simulink model "nmm2DFullBody"  (R2015b)
settings: Solver=ode23s  StartTime=0.0  StopTime=13  FixedStep=1e-3  MaxStep=ts_max  RelTol=1e-3  AbsTol=1e-4
InitFcn:
  | addpath('../lib');
  | addpath('./init_script');
  | nms_model_MechInit
  | nms_model_ControlInit
StopFcn:
  | mRFX = struct;
  | 
  | mRFX.RStance = DataFromModel.Data(:,2)
  | mRFX.RGRF_AP = DataFromModel.Data(:,24)
  | mRFX.RGRF_VT = DataFromModel.Data(:,22)
  | mRFX.RAnkleAngle = DataFromModel.Data(:,8)
  | mRFX.RKneeAngle = DataFromModel.Data(:,7)
  | mRFX.RHipAngle = DataFromModel.Data(:,6)
  | mRFX.RAnkleTorque = DataFromModel.Data(:,20)
  | mRFX.RKneeTorque = DataFromModel.Data(:,19)
  | mRFX.RHipTorque = DataFromModel.Data(:,18)
  | 
  | mRFX.RMuscleGLU = DataFromModel.Data(:,32)
  | mRFX.RMuscleHF = DataFromModel.Data(:,33)
  | mRFX.RMuscleHAM = DataFromModel.Data(:,34)
  | mRFX.RMuscleVAS = DataFromModel.Data(:,35)
  | mRFX.RMuscleGAS = DataFromModel.Data(:,36)
  | mRFX.RMuscleSOL = DataFromModel.Data(:,37)
  | mRFX.RMuscleTA = DataFromModel.Data(:,38)
  | 
  | mRFX.LStance = DataFromModel.Data(:,1)
  | mRFX.LGRF_AP = DataFromModel.Data(:,23)
  | mRFX.LGRF_VT = DataFromModel.Data(:,21)
  | mRFX.LAnkleAngle = DataFromModel.Data(:,5)
  | mRFX.LKneeAngle = DataFromModel.Data(:,4)
  | mRFX.LHipAngle = DataFromModel.Data(:,3)
  | mRFX.LAnkleTorque = DataFromModel.Data(:,17)
  | mRFX.LKneeTorque = DataFromModel.Data(:,16)
  | mRFX.LHipTorque = DataFromModel.Data(:,15)
  | 
  | mRFX.LMuscleGLU = DataFromModel.Data(:,25)
  | mRFX.LMuscleHF = DataFromModel.Data(:,26)
  | mRFX.LMuscleHAM = DataFromModel.Data(:,27)
  | mRFX.LMuscleVAS = DataFromModel.Data(:,28)
  | mRFX.LMuscleGAS = DataFromModel.Data(:,29)
  | mRFX.LMuscleSOL = DataFromModel.Data(:,30)
  | mRFX.LMuscleTA = DataFromModel.Data(:,31)
values from neighbouring files (symbols this model uses):
  c = load('struct_mRFX_HAM_symetric_feedback.mat')    [Ex2b.m]
undefined symbols (not defined in the file or in its folder): alphaFmGas, alphaFmGlu, alphaFmHam, alphaFmSol, alphaFmVas, alphaLceHam, alphaLceHfl, alphaLceTa, alphaLceTa1, Amp, amp_var, c_jointstop, D12_F, D12_S, D12_T, D13_F, D1G_F, D1G_HAT, D1G_S, D1G_T, DeltaThRef, eref, FmaxGAS, FmaxGLU, FmaxHAM, FmaxHFL, FmaxSOL, FmaxTA, FmaxVAS, freq, freq_var, GainDeltaTheta, GainGAS, GainGLU, GainHAM, GainHAMHFL, GainHFL, GainKneOverExt, GainSOL, GainSOLTA, GainTA, GainVAS, In_F, In_HAT, In_S, In_T, K, k_gx, k_gy, k_pressure, K_swing, LceOffsetHAM, LceOffsetHFL, LceOffsetTA, LongDelay, loptGAS, loptGLU, loptHAM, loptHFL, loptSOL ... (+82)
libraries: nmc x77, mblibv1 x60, simulink x33, simulink_extras x18
(part 2 of 8)

== system nmm2DFullBody/Body Mechanics Layer (from Geyer s 2010 model)/Left Ball Contact ==
  note: Planar Ground Interaction Model
  Body Actuator : mblibv1/Sensors &  Actuators/Body Actuator  UpdateFromCAD=off  PhysicalDomain=Mechanical  PortType=blob  ActuationStyle=Force  AngleUnits=deg  ArcVelocityUnits=deg/s  ArcAccelerationUnits=deg/s^2  CoordPositionUnits=m  VelocityUnits=m/s  AccelerationUnits=m/s^2  ForceUnits=N  TorqueUnits=N-m  ActiveIO=on  Width=3  DialogClass=MechanicalActuatorBlock  ReferenceFrame=Absolute (World)  Angle=off  CoordPosition=on  Force=on  Torque=off
  Body Sensor : mblibv1/Sensors &  Actuators/Body Sensor  UpdateFromCAD=off  PhysicalDomain=Mechanical  PortType=blob  Muxed=on  Pose=off  Angle=on  AngleUnits=deg  ArcVelocity=off  ArcVelocityUnits=deg/s  ArcAcceleration=off  ArcAccelerationUnits=deg/s^2  CoordPosition=on  CoordPositionUnits=m  Velocity=on  VelocityUnits=m/s  Acceleration=off  AccelerationUnits=m/s^2  Quaternion=on  QuaternionDT=off  QuaternionDDT=off  QuaternionUnits=off  OutputVector=[ 3 3 ]  ActiveIO=on  Width=6  DialogClass=MechanicalSensorBlock  ReferenceFrame=Absolute (World)
  Demux1 : Demux
  Ground Friction Model : Subsystem
  Ground1 : Ground
  Mechanical Branching Bar : mblibv1/Utilities/Mechanical Branching Bar  LConnTagsString=_newl0  RConnTagsString=SA0|SA1  UpdateFromCAD=off  DialogClass=MechanicalBranchingBarBlock  NumSAPorts=2
  Mux : Mux  Inputs=2
  Mux1 : Mux  Inputs=3
  Sum : Sum  Inputs=-+|
  Terminator : Terminator
  To Workspace : ToWorkspace  VariableName=L_dyvyxvx  SaveFormat=Timeseries  SampleTime=-1
  Vector ConcatenateKnee : Concatenate  NumInputs=4
  "[y y' x x']" : Selector  InputPortWidth=6  IndexOptions=Index vector (dialog)  Indices=[2 5 1 4]  OutputSizes=1
  contact? : simulink/Logic and Bit Operations/Compare To Zero  relop=<=  OutDataTypeStr=boolean
  yGround : Constant  Value=0
  F : PMIOPort  Port=1  Side=Left
  LBallCnt : Outport
  GRF [N N] : Outport  Port=2
  wires:
  contact?/1 -> Ground Friction Model/Enable, LBallCnt/1
  Ground Friction Model/1(Fy_Ground[N]) -> Mux/2, Mux1/2
  Ground Friction Model/2(Fx_Friction [N]) -> Mux/1, Mux1/1
  Ground Friction Model/3(Stiction!) -> Terminator/1
  Mux/1 -> GRF [N N]/1
  yGround/1 -> Sum/1
  Sum/1 -> Vector ConcatenateKnee/1, Ground Friction Model/1(dy [m]), contact?/1
  Body Sensor/1 -> "[y y' x x']"/1
  Mux1/1 -> Body Actuator/1
  Demux1/1 -> Sum/2
  Demux1/2 -> Vector ConcatenateKnee/2, Ground Friction Model/2(vy [m/s])
  Demux1/4 -> Vector ConcatenateKnee/4, Ground Friction Model/4(vx [m/s])
  "[y y' x x']"/1 -> Demux1/1
  Ground1/1 -> Mux1/3
  Vector ConcatenateKnee/1 -> To Workspace/1
  Demux1/3 -> Vector ConcatenateKnee/3, Ground Friction Model/3(x [m])
  connections:
  F/RConn1 -- Mechanical Branching Bar/LConn1
  Mechanical Branching Bar/RConn1 -- Body Sensor/LConn1
  Mechanical Branching Bar/RConn2 -- Body Actuator/RConn1

== system nmm2DFullBody/Body Mechanics Layer (from Geyer s 2010 model)/Left Heel Contact ==
  note: Planar Ground Interaction Model
  Body Actuator : mblibv1/Sensors &  Actuators/Body Actuator  UpdateFromCAD=off  PhysicalDomain=Mechanical  PortType=blob  ActuationStyle=Force  AngleUnits=deg  ArcVelocityUnits=deg/s  ArcAccelerationUnits=deg/s^2  CoordPositionUnits=m  VelocityUnits=m/s  AccelerationUnits=m/s^2  ForceUnits=N  TorqueUnits=N-m  ActiveIO=on  Width=3  DialogClass=MechanicalActuatorBlock  ReferenceFrame=Absolute (World)  Angle=off  CoordPosition=on  Force=on  Torque=off
  Body Sensor : mblibv1/Sensors &  Actuators/Body Sensor  UpdateFromCAD=off  PhysicalDomain=Mechanical  PortType=blob  Muxed=on  Pose=off  Angle=on  AngleUnits=deg  ArcVelocity=off  ArcVelocityUnits=deg/s  ArcAcceleration=off  ArcAccelerationUnits=deg/s^2  CoordPosition=on  CoordPositionUnits=m  Velocity=on  VelocityUnits=m/s  Acceleration=off  AccelerationUnits=m/s^2  Quaternion=on  QuaternionDT=off  QuaternionDDT=off  QuaternionUnits=off  OutputVector=[ 3 3 ]  ActiveIO=on  Width=6  DialogClass=MechanicalSensorBlock  ReferenceFrame=Absolute (World)
  Demux1 : Demux
  Ground Friction Model : Subsystem
  Ground1 : Ground
  Mechanical Branching Bar : mblibv1/Utilities/Mechanical Branching Bar  LConnTagsString=_newl0  RConnTagsString=SA0|SA1  UpdateFromCAD=off  DialogClass=MechanicalBranchingBarBlock  NumSAPorts=2
  Mux : Mux  Inputs=2
  Mux1 : Mux  Inputs=3
  Sum : Sum  Inputs=-+|
  Terminator : Terminator
  "[y y' x x']" : Selector  InputPortWidth=6  IndexOptions=Index vector (dialog)  Indices=[2 5 1 4]  OutputSizes=1
  skin contact sensor : simulink/Logic and Bit Operations/Compare To Zero  relop=<=  OutDataTypeStr=boolean
  yGround : Constant  Value=0
  F : PMIOPort  Port=1  Side=Left
  LHeelCnt : Outport
  GRF [N N] : Outport  Port=2
  wires:
  Ground Friction Model/3(Stiction!) -> Terminator/1
  Ground Friction Model/2(Fx_Friction [N]) -> Mux/1, Mux1/1
  Ground Friction Model/1(Fy_Ground[N]) -> Mux/2, Mux1/2
  skin contact sensor/1 -> Ground Friction Model/Enable, LHeelCnt/1
  Mux/1 -> GRF [N N]/1
  yGround/1 -> Sum/1
  Sum/1 -> Ground Friction Model/1(dy [m]), skin contact sensor/1
  Body Sensor/1 -> "[y y' x x']"/1
  Mux1/1 -> Body Actuator/1
  Demux1/1 -> Sum/2
  Demux1/2 -> Ground Friction Model/2(vy [m/s])
  Demux1/3 -> Ground Friction Model/3(x [m])
  Demux1/4 -> Ground Friction Model/4(vx [m/s])
  "[y y' x x']"/1 -> Demux1/1
  Ground1/1 -> Mux1/3
  connections:
  Mechanical Branching Bar/RConn2 -- Body Actuator/RConn1
  Mechanical Branching Bar/RConn1 -- Body Sensor/LConn1
  F/RConn1 -- Mechanical Branching Bar/LConn1

== system nmm2DFullBody/Body Mechanics Layer (from Geyer s 2010 model)/Left Force Plate ==
  "GRF_Ball [N N] " : Inport
  GRF_Heel [N N] : Inport  Port=2
  Enable : EnablePort  StatesWhenEnabling=reset
  Fcn : Fcn  Expr=u(1)/(u(2)+eps)
  Mux : Mux  Inputs=3
  Mux1 : Mux  Inputs=2
  Selector : Selector  InputPortWidth=2  IndexOptions=Index vector (dialog)  Indices=2  OutputSizes=1
  Selector1 : Selector  InputPortWidth=2  IndexOptions=Index vector (dialog)  Indices=2  OutputSizes=1
  Sum1 : Sum
  GRFs : Outport  OutputWhenDisabled=reset  InitialOutput=0
  COP : Outport  Port=2  OutputWhenDisabled=reset  InitialOutput=0
  wires:
  Selector/1 -> Mux1/2
  Selector1/1 -> Mux1/1
  "GRF_Ball [N N] "/1 -> Sum1/1, Mux/1, Selector1/1
  GRF_Heel [N N]/1 -> Sum1/2, Mux/3
  Sum1/1 -> Mux/2, Selector/1
  Mux/1 -> GRFs/1
  Mux1/1 -> Fcn/1
  Fcn/1 -> COP/1

== system nmm2DFullBody/Body Mechanics Layer (from Geyer s 2010 model)/Left Thigh Sensor Sheet ==
  note: Inner Segment Pressure Sheet
  Gain3 : Gain  Gain=k_pressure
  Gain4 : Gain  Gain=1/v_max_pressure
  Inner Thigh Shift Joint : mblibv1/Joints/Prismatic  LConnTagsString=__newl0|SA1|SA2  RConnTagsString=__newr0|SA1  UpdateFromCAD=off  NumSAPorts=3  CutJoint=off  MarkAsCut=off  Primitives=prismatic  PrimitiveProps=P1$WORLD$[1 0 0]$prismatic  DialogClass=JointBlock  P1Axis=[1 0 0]
  Left Thigh Sensor Sheet IC : mblibv1/Sensors &  Actuators/Joint Initial Condition  UpdateFromCAD=off  LeftPortType=blob  RightPortType=blob  PhysicalDomain=mechanical  DialogClass=InitialConditionBlock  InitialConditions=P1$true$0$m$rad$0$m/s$rad/s#P2$false$0$m$rad$0$m/s$rad/s#P3$false$0$m$rad$0$m/s$rad/s#R1$false$0$m$rad$0$m/s$rad/s#R2$false$0$m$rad$0$m/s$rad/s#R3$false$0$m$rad$0$m/s$rad/s#S$false$0$m$rad$0$m/s$rad/s  P1PIC=0  P1VIC=0  P2PIC=0  P2VIC=0  P3PIC=0  P3VIC=0  R1PIC=0  R1VIC=0  R2PIC=0  R2VIC=0  R3PIC=0  R3VIC=0  SPIC=0  SVIC=0
  Mux1 : Mux  Inputs=2
  Pressure Sheet Reaction Force : Fcn  Expr=-u(1) * (1+sgn(u(1))*u(2))
  Thigh Actuator : mblibv1/Sensors &  Actuators/Joint Actuator  UpdateFromCAD=off  PhysicalDomain=Mechanical  PortType=blob  ActuationStyle=Force  AngleUnits=deg  ArcVelocityUnits=deg/s  ArcAccelerationUnits=deg/s^2  CoordPositionUnits=m  VelocityUnits=m/s  AccelerationUnits=m/s^2  ForceUnits=N  TorqueUnits=N-m  ActiveIO=on  Width=1  DialogClass=MechanicalActuatorBlock  Primitive=P1  ReferenceFrame=Absolute (INERTIAL)
  Thigh Sensor : mblibv1/Sensors &  Actuators/Joint Sensor  UpdateFromCAD=off  PhysicalDomain=Mechanical  PortType=blob  Muxed=off  Pose=off  Angle=on  AngleUnits=deg  ArcVelocity=off  ArcVelocityUnits=deg/s  ArcAcceleration=off  ArcAccelerationUnits=deg/s^2  CoordPosition=on  CoordPositionUnits=m  Velocity=on  VelocityUnits=m/s  Acceleration=off  AccelerationUnits=m/s^2  Quaternion=on  QuaternionDT=off  QuaternionDDT=off  QuaternionUnits=off  OutputVector=[ 1 1 ]  ActiveIO=on  Width=2  DialogClass=MechanicalSensorBlock  Primitive=P1  Force=off  ForceUnits=N  Torque=off  TorqueUnits=N-m  ReferenceFrame=Absolute (INERTIAL)  ReactionSensedSide=Base  ReactionReferenceFrame=Absolute (World)  ReactionForce=off  ReactionForceUnits=N  ReactionMoment=off  ReactionMomentUnits=N-m
  B : PMIOPort  Tag=PMCPort  Port=1  Side=Left
  F : PMIOPort  Tag=PMCPort  Port=2  Side=Right
  dx : Outport
  wires:
  Thigh Sensor/1 -> Gain3/1, dx/1
  Thigh Sensor/2 -> Gain4/1
  Mux1/1 -> Pressure Sheet Reaction Force/1
  Gain3/1 -> Mux1/1
  Gain4/1 -> Mux1/2
  Pressure Sheet Reaction Force/1 -> Thigh Actuator/1
  connections:
  B/RConn1 -- Inner Thigh Shift Joint/LConn1
  F/RConn1 -- Inner Thigh Shift Joint/RConn1
  Thigh Sensor/LConn1 -- Inner Thigh Shift Joint/LConn2
  Inner Thigh Shift Joint/RConn2 -- Thigh Actuator/RConn1
  Left Thigh Sensor Sheet IC/RConn1 -- Inner Thigh Shift Joint/LConn3

== system nmm2DFullBody/Body Mechanics Layer (from Geyer s 2010 model)/Right Ball Contact ==
  note: Planar Ground Interaction Model
  Body Actuator : mblibv1/Sensors &  Actuators/Body Actuator  UpdateFromCAD=off  PhysicalDomain=Mechanical  PortType=blob  ActuationStyle=Force  AngleUnits=deg  ArcVelocityUnits=deg/s  ArcAccelerationUnits=deg/s^2  CoordPositionUnits=m  VelocityUnits=m/s  AccelerationUnits=m/s^2  ForceUnits=N  TorqueUnits=N-m  ActiveIO=on  Width=3  DialogClass=MechanicalActuatorBlock  ReferenceFrame=Absolute (World)  Angle=off  CoordPosition=on  Force=on  Torque=off
  Body Sensor : mblibv1/Sensors &  Actuators/Body Sensor  UpdateFromCAD=off  PhysicalDomain=Mechanical  PortType=blob  Muxed=on  Pose=off  Angle=on  AngleUnits=deg  ArcVelocity=off  ArcVelocityUnits=deg/s  ArcAcceleration=off  ArcAccelerationUnits=deg/s^2  CoordPosition=on  CoordPositionUnits=m  Velocity=on  VelocityUnits=m/s  Acceleration=off  AccelerationUnits=m/s^2  Quaternion=on  QuaternionDT=off  QuaternionDDT=off  QuaternionUnits=off  OutputVector=[ 3 3 ]  ActiveIO=on  Width=6  DialogClass=MechanicalSensorBlock  ReferenceFrame=Absolute (World)
  Demux1 : Demux
  Ground : Ground
  Ground Friction Model : Subsystem
  Mechanical Branching Bar : mblibv1/Utilities/Mechanical Branching Bar  LConnTagsString=_newl0  RConnTagsString=SA0|SA1  UpdateFromCAD=off  DialogClass=MechanicalBranchingBarBlock  NumSAPorts=2
  Mux : Mux  Inputs=2
  Mux1 : Mux  Inputs=3
  Sum : Sum  Inputs=-+|
  Terminator : Terminator
  To Workspace : ToWorkspace  VariableName=R_dyvyxvx  SaveFormat=Timeseries  SampleTime=-1
  Vector ConcatenateKnee : Concatenate  NumInputs=4
  "[y y' x x']" : Selector  InputPortWidth=6  IndexOptions=Index vector (dialog)  Indices=[2 5 1 4]  OutputSizes=1
  contact? : simulink/Logic and Bit Operations/Compare To Zero  relop=<=  OutDataTypeStr=boolean
  yGround : Constant  Value=0
  F : PMIOPort  Port=1  Side=Left
  RBallCnt : Outport
  GRF [N N] : Outport  Port=2
  wires:
  Demux1/2 -> Vector ConcatenateKnee/2, Ground Friction Model/2(vy [m/s])
  contact?/1 -> Ground Friction Model/Enable, RBallCnt/1
  Ground Friction Model/1(Fy_Ground[N]) -> Mux/2, Mux1/2
  Ground Friction Model/2(Fx_Friction [N]) -> Mux/1, Mux1/1
  Ground Friction Model/3(Stiction!) -> Terminator/1
  Mux/1 -> GRF [N N]/1
  Sum/1 -> Vector ConcatenateKnee/1, Ground Friction Model/1(dy [m]), contact?/1
  yGround/1 -> Sum/1
  Body Sensor/1 -> "[y y' x x']"/1
  "[y y' x x']"/1 -> Demux1/1
  Demux1/1 -> Sum/2
  Demux1/3 -> Vector ConcatenateKnee/3, Ground Friction Model/3(x [m])
  Demux1/4 -> Vector ConcatenateKnee/4, Ground Friction Model/4(vx [m/s])
  Ground/1 -> Mux1/3
  Mux1/1 -> Body Actuator/1
  Vector ConcatenateKnee/1 -> To Workspace/1
  connections:
  F/RConn1 -- Mechanical Branching Bar/LConn1
  Mechanical Branching Bar/RConn2 -- Body Actuator/RConn1
  Mechanical Branching Bar/RConn1 -- Body Sensor/LConn1

== system nmm2DFullBody/Body Mechanics Layer (from Geyer s 2010 model)/Right Heel Contact ==
  note: Planar Ground Interaction Model
  Body Actuator : mblibv1/Sensors &  Actuators/Body Actuator  UpdateFromCAD=off  PhysicalDomain=Mechanical  PortType=blob  ActuationStyle=Force  AngleUnits=deg  ArcVelocityUnits=deg/s  ArcAccelerationUnits=deg/s^2  CoordPositionUnits=m  VelocityUnits=m/s  AccelerationUnits=m/s^2  ForceUnits=N  TorqueUnits=N-m  ActiveIO=on  Width=3  DialogClass=MechanicalActuatorBlock  ReferenceFrame=Absolute (World)  Angle=off  CoordPosition=on  Force=on  Torque=off
  Body Sensor : mblibv1/Sensors &  Actuators/Body Sensor  UpdateFromCAD=off  PhysicalDomain=Mechanical  PortType=blob  Muxed=on  Pose=off  Angle=on  AngleUnits=deg  ArcVelocity=off  ArcVelocityUnits=deg/s  ArcAcceleration=off  ArcAccelerationUnits=deg/s^2  CoordPosition=on  CoordPositionUnits=m  Velocity=on  VelocityUnits=m/s  Acceleration=off  AccelerationUnits=m/s^2  Quaternion=on  QuaternionDT=off  QuaternionDDT=off  QuaternionUnits=off  OutputVector=[ 3 3 ]  ActiveIO=on  Width=6  DialogClass=MechanicalSensorBlock  ReferenceFrame=Absolute (World)
  Demux1 : Demux
  Ground : Ground
  Ground Friction Model : Subsystem
  Mechanical Branching Bar : mblibv1/Utilities/Mechanical Branching Bar  LConnTagsString=_newl0  RConnTagsString=SA0|SA1  UpdateFromCAD=off  DialogClass=MechanicalBranchingBarBlock  NumSAPorts=2
  Mux : Mux  Inputs=2
  Mux1 : Mux  Inputs=3
  Sum : Sum  Inputs=-+|
  Terminator : Terminator
  "[y y' x x']" : Selector  InputPortWidth=6  IndexOptions=Index vector (dialog)  Indices=[2 5 1 4]  OutputSizes=1
  contact? : simulink/Logic and Bit Operations/Compare To Zero  relop=<=  OutDataTypeStr=boolean
  yGround : Constant  Value=0
  F : PMIOPort  Port=1  Side=Left
  RHeelCnt : Outport
  GRF [N N] : Outport  Port=2
  wires:
  Ground Friction Model/3(Stiction!) -> Terminator/1
  Ground Friction Model/2(Fx_Friction [N]) -> Mux/1, Mux1/1
  Ground Friction Model/1(Fy_Ground[N]) -> Mux/2, Mux1/2
  contact?/1 -> Ground Friction Model/Enable, RHeelCnt/1
  Demux1/4 -> Ground Friction Model/4(vx [m/s])
  Demux1/3 -> Ground Friction Model/3(x [m])
  Demux1/2 -> Ground Friction Model/2(vy [m/s])
  Mux/1 -> GRF [N N]/1
  yGround/1 -> Sum/1
  Demux1/1 -> Sum/2  "yBall"
  Sum/1 -> Ground Friction Model/1(dy [m]), contact?/1
  Body Sensor/1 -> "[y y' x x']"/1
  "[y y' x x']"/1 -> Demux1/1
  Mux1/1 -> Body Actuator/1
  Ground/1 -> Mux1/3
  connections:
  F/RConn1 -- Mechanical Branching Bar/LConn1
  Mechanical Branching Bar/RConn1 -- Body Sensor/LConn1
  Mechanical Branching Bar/RConn2 -- Body Actuator/RConn1

== system nmm2DFullBody/Body Mechanics Layer (from Geyer s 2010 model)/Right Force Plate ==
  "GRF_Ball [N N] " : Inport
  GRF_Heel [N N] : Inport  Port=2
  Enable : EnablePort  StatesWhenEnabling=reset
  Fcn : Fcn  Expr=u(1)/(u(2)+eps)
  Mux : Mux  Inputs=3
  Mux1 : Mux  Inputs=2
  Selector : Selector  InputPortWidth=2  IndexOptions=Index vector (dialog)  Indices=2  OutputSizes=1
  Selector1 : Selector  InputPortWidth=2  IndexOptions=Index vector (dialog)  Indices=2  OutputSizes=1
  Sum1 : Sum
  GRFs : Outport  OutputWhenDisabled=reset  InitialOutput=0
  COP : Outport  Port=2  OutputWhenDisabled=reset  InitialOutput=0
  wires:
  Selector/1 -> Mux1/2
  Selector1/1 -> Mux1/1
  "GRF_Ball [N N] "/1 -> Sum1/1, Mux/1, Selector1/1
  GRF_Heel [N N]/1 -> Sum1/2, Mux/3
  Sum1/1 -> Mux/2, Selector/1
  Mux/1 -> GRFs/1
  Mux1/1 -> Fcn/1
  Fcn/1 -> COP/1

== system nmm2DFullBody/Body Mechanics Layer (from Geyer s 2010 model)/Right Thigh Sensor Sheet ==
  note: Inner Segment Pressure Sheet
  Gain3 : Gain  Gain=k_pressure
  Gain4 : Gain  Gain=1/v_max_pressure
  Inner Thigh Shift Joint : mblibv1/Joints/Prismatic  LConnTagsString=__newl0|SA1|SA2  RConnTagsString=__newr0|SA1  UpdateFromCAD=off  NumSAPorts=3  CutJoint=off  MarkAsCut=off  Primitives=prismatic  PrimitiveProps=P1$WORLD$[1 0 0]$prismatic  DialogClass=JointBlock  P1Axis=[1 0 0]
  Mux1 : Mux  Inputs=2
  Pressure Sheet Reaction Force : Fcn  Expr=-u(1) * (1+sgn(u(1))*u(2))
  Right Thigh Sensor Sheet IC : mblibv1/Sensors &  Actuators/Joint Initial Condition  UpdateFromCAD=off  LeftPortType=blob  RightPortType=blob  PhysicalDomain=mechanical  DialogClass=InitialConditionBlock  InitialConditions=P1$true$0$m$rad$0$m/s$rad/s#P2$false$0$m$rad$0$m/s$rad/s#P3$false$0$m$rad$0$m/s$rad/s#R1$false$0$m$rad$0$m/s$rad/s#R2$false$0$m$rad$0$m/s$rad/s#R3$false$0$m$rad$0$m/s$rad/s#S$false$0$m$rad$0$m/s$rad/s  P1PIC=0  P1VIC=0  P2PIC=0  P2VIC=0  P3PIC=0  P3VIC=0  R1PIC=0  R1VIC=0  R2PIC=0  R2VIC=0  R3PIC=0  R3VIC=0  SPIC=0  SVIC=0
  Thigh Actuator : mblibv1/Sensors &  Actuators/Joint Actuator  UpdateFromCAD=off  PhysicalDomain=Mechanical  PortType=blob  ActuationStyle=Force  AngleUnits=deg  ArcVelocityUnits=deg/s  ArcAccelerationUnits=deg/s^2  CoordPositionUnits=m  VelocityUnits=m/s  AccelerationUnits=m/s^2  ForceUnits=N  TorqueUnits=N-m  ActiveIO=on  Width=1  DialogClass=MechanicalActuatorBlock  Primitive=P1  ReferenceFrame=Absolute (INERTIAL)
  Thigh Sensor : mblibv1/Sensors &  Actuators/Joint Sensor  UpdateFromCAD=off  PhysicalDomain=Mechanical  PortType=blob  Muxed=off  Pose=off  Angle=on  AngleUnits=deg  ArcVelocity=off  ArcVelocityUnits=deg/s  ArcAcceleration=off  ArcAccelerationUnits=deg/s^2  CoordPosition=on  CoordPositionUnits=m  Velocity=on  VelocityUnits=m/s  Acceleration=off  AccelerationUnits=m/s^2  Quaternion=on  QuaternionDT=off  QuaternionDDT=off  QuaternionUnits=off  OutputVector=[ 1 1 ]  ActiveIO=on  Width=2  DialogClass=MechanicalSensorBlock  Primitive=P1  Force=off  ForceUnits=N  Torque=off  TorqueUnits=N-m  ReferenceFrame=Absolute (INERTIAL)  ReactionSensedSide=Base  ReactionReferenceFrame=Absolute (World)  ReactionForce=off  ReactionForceUnits=N  ReactionMoment=off  ReactionMomentUnits=N-m
  B : PMIOPort  Tag=PMCPort  Port=1  Side=Left
  F : PMIOPort  Tag=PMCPort  Port=2  Side=Right
  dx : Outport
  wires:
  Thigh Sensor/1 -> Gain3/1, dx/1
  Thigh Sensor/2 -> Gain4/1
  Mux1/1 -> Pressure Sheet Reaction Force/1
  Gain3/1 -> Mux1/1
  Gain4/1 -> Mux1/2
  Pressure Sheet Reaction Force/1 -> Thigh Actuator/1
  connections:
  B/RConn1 -- Inner Thigh Shift Joint/LConn1
  F/RConn1 -- Inner Thigh Shift Joint/RConn1
  Thigh Sensor/LConn1 -- Inner Thigh Shift Joint/LConn2
  Inner Thigh Shift Joint/RConn2 -- Thigh Actuator/RConn1
  Inner Thigh Shift Joint/LConn3 -- Right Thigh Sensor Sheet IC/RConn1

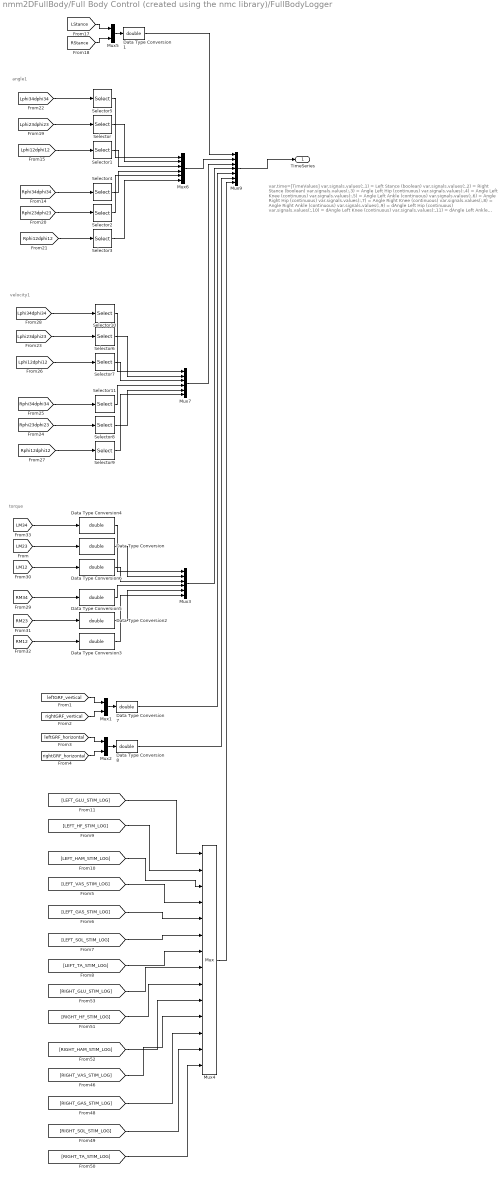
== system nmm2DFullBody/Full Body Control (created using the nmc library)/FullBodyLogger ==
  note: torque
  note: velocity1
  note: angle1
  note: var.time=[TimeValues]
      | var.signals.values(:,1) = Left Stance (boolean)
      | var.signals.values(:,2) = Right Stance (boolean)
      | var.signals.values(:,3) = Angle Left Hip (continuous)
      | var.signals.values(:,4) = Angle Left Knee (continuous)
      | var.signals.values(:,5) = Angle Left Ankle (continuous)
      | var.signals.values(:,6) = Angle Right Hip (continuous)
      | var.signals.values(:,7) = Angle Right Knee (continuous)
      | var.signals.values(:,8) = Angle Right Ankle (continuous)
      | var.signals.values(:,9) = dAngle Left Hip (continuous)
      | var.signals.values(:,10) = dAngle Left Knee (continuous)
      | var.signals.values(:,11) = dAngle Left Ankle (continuous)
      | var.signals.values(:,12) = dAngle Right Hip (continuous)
      | var.signals.values(:,13) = dAngle Right Knee (continuous)
      | var.signals.values(:,14) = dAngle Right Ankle (continuous)
      | var.signals.values(:,15) = Torque Left Hip (continuous)
      | var.signals.values(:,16) = Torque Left Knee (continuous)
      | var.signals.values(:,17) = Torque Left Ankle (continuous)
      | var.signals.values(:,18) = Torque Right Hip (continuous)
      | var.signals.values(:,19) = Torque Right Knee (continuous)
      | var.signals.values(:,20) = Torque Right Ankle (continuous)
      | var.signals.values(:,21) = Force Left vGRF (continuous)
      | var.signals.values(:,22) = Force Right vGRF (continuous)
      | var.signals.values(:,23) = Force Left hGRF (continuous)
      | var.signals.values(:,24) = Force Right hGRF (continuous)
      | var.signals.values(:,25) = GLU (left continous)
      | var.signals.values(:,26) = HF (left continous)
      | var.signals.values(:,27) = HAM (left continous)
      | var.signals.values(:,28) = VAS (left continous)
      | var.signals.values(:,29) = GAS (left continous)
      | var.signals.values(:,30) = SOL (left continous)
      | var.signals.values(:,31) = TA (left continous)
      | var.signals.values(:,32) = GLU (right continous)
      | var.signals.values(:,33) = HF (right continous)
      | var.signals.values(:,34) = HAM (right continous)
      | var.signals.values(:,35) = VAS (right continous)
      | var.signals.values(:,36) = GAS (right continous)
      | var.signals.values(:,37) = SOL (right continous)
      | var.signals.values(:,38) = TA (right continous)
      | var.signals.dimensions=[38]
  Data Type Conversion{,1..8} (9 alike) : DataTypeConversion  OutDataTypeStr=double
  Mux1 : Mux  Inputs=2
  Mux2 : Mux  Inputs=2
  Mux3 : Mux  Inputs=6
  Mux4 : Mux  Inputs=14
  Mux5 : Mux  Inputs=2
  Mux6 : Mux  Inputs=6
  Mux7 : Mux  Inputs=6
  Mux9 : Mux  Inputs=7
  Selector{,1..5} (6 alike) : Selector  InputPortWidth=2  IndexOptions=Index vector (dialog)  Indices=[1]  OutputSizes=1
  Selector{6..11} (6 alike) : Selector  InputPortWidth=2  IndexOptions=Index vector (dialog)  Indices=[2]  OutputSizes=1
  TimeSeries : Outport
  wires:
  [Rphi34dphi34] -> Selector4/1
  [Lphi34dphi34] -> Selector10/1
  Selector11/1 -> Mux7/4
  [Rphi34dphi34] -> Selector11/1
  [LM12] -> Data Type Conversion6/1
  [RM23] -> Data Type Conversion2/1
  Data Type Conversion3/1 -> Mux3/6
  [RM34] -> Data Type Conversion5/1
  Selector5/1 -> Mux6/1
  Selector4/1 -> Mux6/4
  [LM23] -> Data Type Conversion/1
  Selector10/1 -> Mux7/1
  Data Type Conversion2/1 -> Mux3/5
  Data Type Conversion/1 -> Mux3/2
  [Lphi12dphi12] -> Selector1/1
  [Rphi12dphi12] -> Selector3/1
  [RM12] -> Data Type Conversion3/1
  [LM34] -> Data Type Conversion4/1
  Data Type Conversion4/1 -> Mux3/1
  [Lphi23dphi23] -> Selector/1
  [Rphi23dphi23] -> Selector2/1
  Selector3/1 -> Mux6/6
  Selector6/1 -> Mux7/2
  Selector7/1 -> Mux7/3
  Mux3/1 -> Mux9/4
  Selector8/1 -> Mux7/5
  Selector9/1 -> Mux7/6
  Mux5/1 -> Data Type Conversion1/1
  Mux6/1 -> Mux9/2
  Mux7/1 -> Mux9/3
  Data Type Conversion1/1 -> Mux9/1
  Mux9/1 -> TimeSeries/1
  [Lphi34dphi34] -> Selector5/1
  [Lphi12dphi12] -> Selector7/1
  [Lphi23dphi23] -> Selector6/1
  [Rphi12dphi12] -> Selector9/1
  [Rphi23dphi23] -> Selector8/1
  [LStance] -> Mux5/1
  [RStance] -> Mux5/2
  Selector/1 -> Mux6/2
  Selector2/1 -> Mux6/5
  Selector1/1 -> Mux6/3
  Data Type Conversion5/1 -> Mux3/4
  Data Type Conversion6/1 -> Mux3/3
  [leftGRF_vertical] -> Mux1/1
  [rightGRF_vertical] -> Mux1/2
  Mux1/1 -> Data Type Conversion7/1
  Data Type Conversion7/1 -> Mux9/5
  [leftGRF_horizontal] -> Mux2/1
  [rightGRF_horizontal] -> Mux2/2
  Mux2/1 -> Data Type Conversion8/1
  Data Type Conversion8/1 -> Mux9/6
  [LEFT_GLU_STIM_LOG] -> Mux4/1
  [LEFT_HF_STIM_LOG] -> Mux4/2
  [LEFT_HAM_STIM_LOG] -> Mux4/3
  [LEFT_VAS_STIM_LOG] -> Mux4/4
  [LEFT_GAS_STIM_LOG] -> Mux4/5
  [LEFT_SOL_STIM_LOG] -> Mux4/6
  [LEFT_TA_STIM_LOG] -> Mux4/7
  [RIGHT_GLU_STIM_LOG] -> Mux4/8
  [RIGHT_HF_STIM_LOG] -> Mux4/9
  [RIGHT_HAM_STIM_LOG] -> Mux4/10
  [RIGHT_VAS_STIM_LOG] -> Mux4/11
  [RIGHT_GAS_STIM_LOG] -> Mux4/12
  [RIGHT_SOL_STIM_LOG] -> Mux4/13
  [RIGHT_TA_STIM_LOG] -> Mux4/14
  Mux4/1 -> Mux9/7

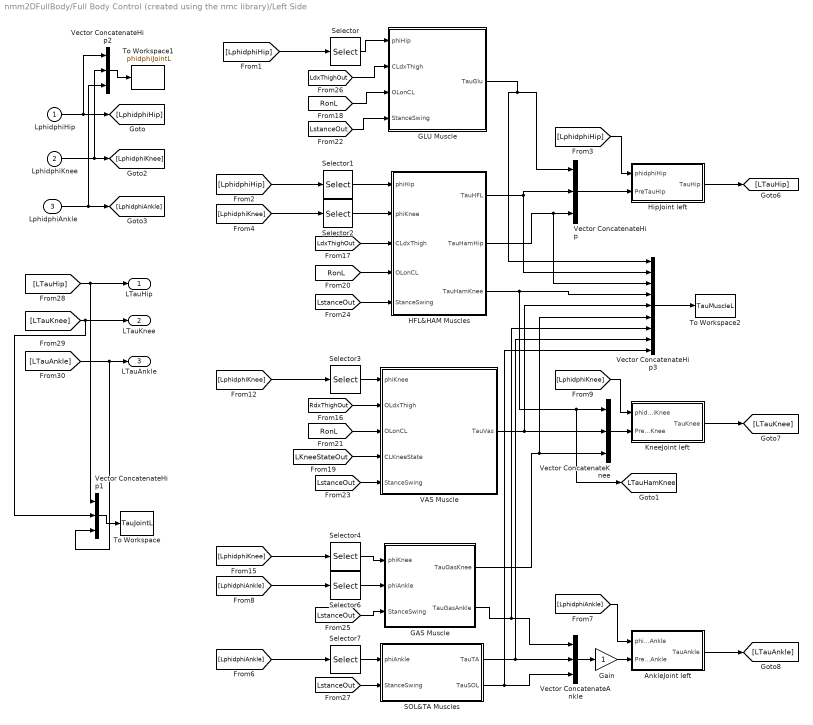
== system nmm2DFullBody/Full Body Control (created using the nmc library)/Left Side ==
  LphidphiHip : Inport
  LphidphiKnee : Inport  Port=2
  LphidphiAnkle : Inport  Port=3
  AnkleJoint left : Subsystem
  GAS Muscle : Subsystem  AncestorBlock=nmc/NMC Muscles/GAS Muscle  mask{VariableName=StimGASL}
      mask prompts: VariableName "Simulink:blkprm_prompts:ToWksVarName"
      mask TypeOptions VariableName: StimGAS/VariableName
  GLU Muscle : Subsystem  AncestorBlock=nmc/NMC Muscles/GLU Muscle  mask{StimGluSide=StimGLU1}
      mask prompts: StimGluSide "Simulink:blkprm_prompts:ToWksVarName"
      mask TypeOptions StimGluSide: StimGLU/VariableName
  Gain : Gain
  HFL&HAM Muscles : Subsystem  AncestorBlock=nmc/NMC Muscles/HFL&HAM Muscles  mask{StimHAMSide=StimHAM, StimHFLSide=StimHFL}
      mask prompts: StimHAMSide "Simulink:blkprm_prompts:ToWksVarName"; StimHFLSide "Simulink:blkprm_prompts:ToWksVarName"
      mask TypeOptions StimHAMSide: StimHAM/VariableName
      mask TypeOptions StimHFLSide: StimHFL/VariableName
  HipJoint left : Subsystem
  KneeJoint left : Subsystem
  SOL&TA Muscles : Subsystem  AncestorBlock=nmc/NMC Muscles/SOL&TA Muscles  mask{VariableName=StimSOLL, VariableNameTA=StimTAL}
      mask prompts: VariableName "Simulink:blkprm_prompts:ToWksVarName"; VariableNameTA "Simulink:blkprm_prompts:ToWksVarName"
      mask TypeOptions VariableName: StimSOL/VariableName
      mask TypeOptions VariableNameTA: StimTA/VariableName
  Selector{,1..4,6..7} (7 alike) : Selector  InputPortWidth=2  IndexOptions=Index vector (dialog)  Indices=[1 ]  OutputSizes=1
  To Workspace : ToWorkspace  VariableName=TauJointL  SaveFormat=Timeseries  SampleTime=-1
  To Workspace1 : ToWorkspace  VariableName=phidphiJointL  SaveFormat=Timeseries  SampleTime=-1
  To Workspace2 : ToWorkspace  VariableName=TauMuscleL  SaveFormat=Timeseries  SampleTime=-1
  VAS Muscle : Subsystem  AncestorBlock=nmc/NMC Muscles/VAS Muscle  mask{VariableName=StimVAS}
      mask prompts: VariableName "Simulink:blkprm_prompts:ToWksVarName"
      mask TypeOptions VariableName: StimVAS/VariableName
  Vector ConcatenateAnkle : Concatenate  NumInputs=3
  Vector ConcatenateHip : Concatenate  NumInputs=3
  Vector ConcatenateHip1 : Concatenate  NumInputs=3
  Vector ConcatenateHip2 : Concatenate  NumInputs=3
  Vector ConcatenateHip3 : Concatenate  NumInputs=9
  Vector ConcatenateKnee : Concatenate  NumInputs=3
  LTauHip : Outport
  LTauKnee : Outport  Port=2
  LTauAnkle : Outport  Port=3
  tag scope: LTauHamKnee=global
  wires:
  HFL&HAM Muscles/3(TauHamKnee) -> Vector ConcatenateHip3/4, [LTauHamKnee], Vector ConcatenateKnee/1
  [LstanceOut] -> SOL&TA Muscles/2(StanceSwing)
  Selector7/1 -> SOL&TA Muscles/1(phiAnkle)
  GLU Muscle/1(TauGlu) -> Vector ConcatenateHip/1, Vector ConcatenateHip3/1
  Vector ConcatenateHip3/1 -> To Workspace2/1
  [LTauKnee] -> Vector ConcatenateHip1/2, LTauKnee/1
  Vector ConcatenateHip2/1 -> To Workspace1/1
  Vector ConcatenateHip1/1 -> To Workspace/1
  [LTauAnkle] -> LTauAnkle/1, Vector ConcatenateHip1/3
  [LTauHip] -> LTauHip/1, Vector ConcatenateHip1/1
  LphidphiAnkle/1 -> [LphidphiAnkle], Vector ConcatenateHip2/3
  LphidphiKnee/1 -> [LphidphiKnee], Vector ConcatenateHip2/2
  LphidphiHip/1 -> [LphidphiHip], Vector ConcatenateHip2/1
  [LdxThighOut] -> HFL&HAM Muscles/3(CLdxThigh)
  [RonL] -> GLU Muscle/3(OLonCL)
  [LstanceOut] -> GLU Muscle/4(StanceSwing)
  [LdxThighOut] -> GLU Muscle/2(CLdxThigh)
  AnkleJoint left/1(TauAnkle) -> [LTauAnkle]
  KneeJoint left/1(TauKnee) -> [LTauKnee]
  HipJoint left/1(TauHip) -> [LTauHip]
  [LphidphiKnee] -> Selector2/1
  [LphidphiHip] -> HipJoint left/1(phidphiHip)
  [LphidphiHip] -> Selector/1
  [LstanceOut] -> VAS Muscle/5(StanceSwing)
  [LphidphiHip] -> Selector1/1
  [LphidphiAnkle] -> Selector6/1
  Selector2/1 -> HFL&HAM Muscles/2(phiKnee)
  HFL&HAM Muscles/2(TauHamHip) -> Vector ConcatenateHip/3, Vector ConcatenateHip3/3
  [LphidphiAnkle] -> Selector7/1
  [LstanceOut] -> GAS Muscle/3(StanceSwing)
  Selector/1 -> GLU Muscle/1(phiHip)
  [LKneeStateOut] -> VAS Muscle/4(CLKneeState)
  [RonL] -> HFL&HAM Muscles/4(OLonCL)
  [LphidphiKnee] -> Selector4/1
  [LphidphiKnee] -> Selector3/1
  [RonL] -> VAS Muscle/3(OLonCL)
  [LstanceOut] -> HFL&HAM Muscles/5(StanceSwing)
  HFL&HAM Muscles/1(TauHFL) -> Vector ConcatenateHip3/2, Vector ConcatenateHip/2
  GAS Muscle/1(TauGasKnee) -> Vector ConcatenateKnee/3, Vector ConcatenateHip3/6
  [LphidphiAnkle] -> AnkleJoint left/1(phidphiAnkle)
  VAS Muscle/1(TauVas) -> Vector ConcatenateKnee/2, Vector ConcatenateHip3/5
  Selector6/1 -> GAS Muscle/2(phiAnkle)
  Selector3/1 -> VAS Muscle/1(phiKnee)
  SOL&TA Muscles/1(TauTA) -> Vector ConcatenateAnkle/2, Vector ConcatenateHip3/8
  Vector ConcatenateKnee/1 -> KneeJoint left/2(PreTauKnee)
  Vector ConcatenateAnkle/1 -> Gain/1
  SOL&TA Muscles/2(TauSOL) -> Vector ConcatenateAnkle/3, Vector ConcatenateHip3/9
  [RdxThighOut] -> VAS Muscle/2(OLdxThigh)
  Selector4/1 -> GAS Muscle/1(phiKnee)
  Selector1/1 -> HFL&HAM Muscles/1(phiHip)
  [LphidphiKnee] -> KneeJoint left/1(phidphiKnee)
  Vector ConcatenateHip/1 -> HipJoint left/2(PreTauHip)
  GAS Muscle/2(TauGasAnkle) -> Vector ConcatenateAnkle/1, Vector ConcatenateHip3/7
  Gain/1 -> AnkleJoint left/2(PreTauAnkle)

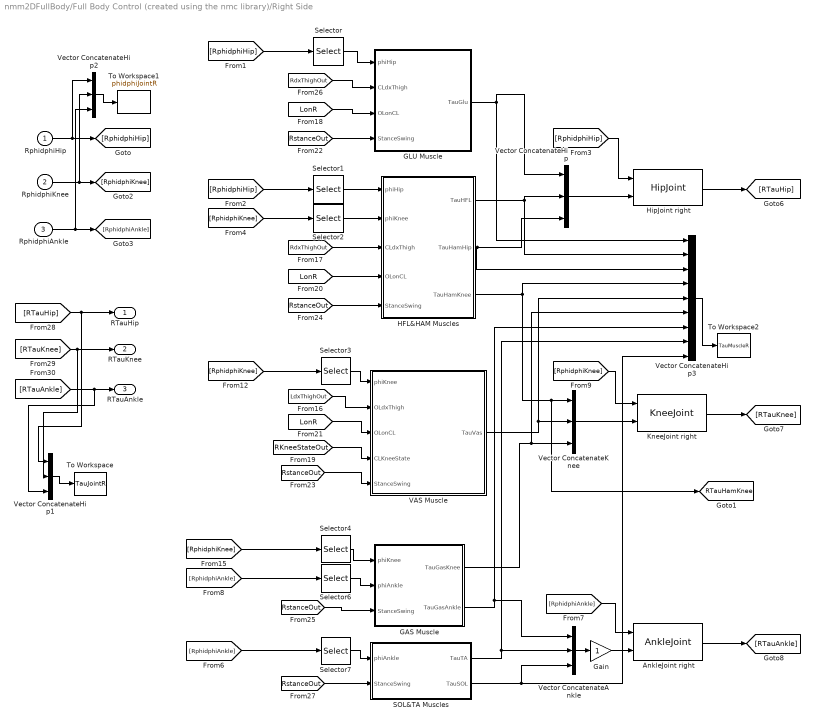
== system nmm2DFullBody/Full Body Control (created using the nmc library)/Right Side ==
  RphidphiHip : Inport
  RphidphiKnee : Inport  Port=2
  RphidphiAnkle : Inport  Port=3
  AnkleJoint right : nmc/NMC Joints/AnkleJoint
  GAS Muscle : Subsystem  AncestorBlock=nmc/NMC Muscles/GAS Muscle  mask{VariableName=StimGASR}
      mask prompts: VariableName "Simulink:blkprm_prompts:ToWksVarName"
      mask TypeOptions VariableName: StimGAS/VariableName
  GLU Muscle : Subsystem  AncestorBlock=nmc/NMC Muscles/GLU Muscle  mask{StimGluSide=StimGLUR}
      mask prompts: StimGluSide "Simulink:blkprm_prompts:ToWksVarName"
      mask TypeOptions StimGluSide: StimGLU/VariableName
  Gain : Gain
  HFL&HAM Muscles : Subsystem  AncestorBlock=nmc/NMC Muscles/HFL&HAM Muscles  mask{StimHAMSide=StimHAMR, StimHFLSide=StimHFLR}
      mask prompts: StimHAMSide "Simulink:blkprm_prompts:ToWksVarName"; StimHFLSide "Simulink:blkprm_prompts:ToWksVarName"
      mask TypeOptions StimHAMSide: StimHAM/VariableName
      mask TypeOptions StimHFLSide: StimHFL/VariableName
  HipJoint right : nmc/NMC Joints/HipJoint
  KneeJoint right : nmc/NMC Joints/KneeJoint
  SOL&TA Muscles : Subsystem  AncestorBlock=nmc/NMC Muscles/SOL&TA Muscles  mask{VariableName=StimSOLR, VariableNameTA=StimTAR}
      mask prompts: VariableName "Simulink:blkprm_prompts:ToWksVarName"; VariableNameTA "Simulink:blkprm_prompts:ToWksVarName"
      mask TypeOptions VariableName: StimSOL/VariableName
      mask TypeOptions VariableNameTA: StimTA/VariableName
  Selector{,1..4,6..7} (7 alike) : Selector  InputPortWidth=2  IndexOptions=Index vector (dialog)  Indices=[1 ]  OutputSizes=1
  To Workspace : ToWorkspace  VariableName=TauJointR  SaveFormat=Timeseries  SampleTime=-1
  To Workspace1 : ToWorkspace  VariableName=phidphiJointR  SaveFormat=Timeseries  SampleTime=-1
  To Workspace2 : ToWorkspace  VariableName=TauMuscleR  SaveFormat=Timeseries  SampleTime=-1
  VAS Muscle : Subsystem  AncestorBlock=nmc/NMC Muscles/VAS Muscle  mask{VariableName=StimVASR}
      mask prompts: VariableName "Simulink:blkprm_prompts:ToWksVarName"
      mask TypeOptions VariableName: StimVAS/VariableName
  Vector ConcatenateAnkle : Concatenate  NumInputs=3
  Vector ConcatenateHip : Concatenate  NumInputs=3
  Vector ConcatenateHip1 : Concatenate  NumInputs=3
  Vector ConcatenateHip2 : Concatenate  NumInputs=3
  Vector ConcatenateHip3 : Concatenate  NumInputs=9
  Vector ConcatenateKnee : Concatenate  NumInputs=3
  RTauHip : Outport
  RTauKnee : Outport  Port=2
  RTauAnkle : Outport  Port=3
  tag scope: RTauHamKnee=global
  wires:
  Vector ConcatenateHip3/1 -> To Workspace2/1
  Vector ConcatenateHip2/1 -> To Workspace1/1
  Vector ConcatenateHip1/1 -> To Workspace/1
  [RTauAnkle] -> RTauAnkle/1, Vector ConcatenateHip1/3
  [RTauKnee] -> RTauKnee/1, Vector ConcatenateHip1/2
  [RTauHip] -> RTauHip/1, Vector ConcatenateHip1/1
  RphidphiAnkle/1 -> Vector ConcatenateHip2/3, [RphidphiAnkle]
  RphidphiKnee/1 -> [RphidphiKnee], Vector ConcatenateHip2/2
  RphidphiHip/1 -> [RphidphiHip], Vector ConcatenateHip2/1
  [RstanceOut] -> HFL&HAM Muscles/5(StanceSwing)
  [LonR] -> HFL&HAM Muscles/4(OLonCL)
  [RdxThighOut] -> HFL&HAM Muscles/3(CLdxThigh)
  [RstanceOut] -> GLU Muscle/4(StanceSwing)
  [LonR] -> GLU Muscle/3(OLonCL)
  [RdxThighOut] -> GLU Muscle/2(CLdxThigh)
  AnkleJoint right/1 -> [RTauAnkle]
  KneeJoint right/1 -> [RTauKnee]
  HipJoint right/1 -> [RTauHip]
  [RphidphiKnee] -> Selector2/1
  [RphidphiHip] -> HipJoint right/1
  [RphidphiHip] -> Selector/1
  [RstanceOut] -> VAS Muscle/5(StanceSwing)
  [RphidphiHip] -> Selector1/1
  [RphidphiAnkle] -> Selector6/1
  Selector2/1 -> HFL&HAM Muscles/2(phiKnee)
  HFL&HAM Muscles/2(TauHamHip) -> Vector ConcatenateHip/3, Vector ConcatenateHip3/3
  [RstanceOut] -> SOL&TA Muscles/2(StanceSwing)
  [RphidphiAnkle] -> Selector7/1
  [RstanceOut] -> GAS Muscle/3(StanceSwing)
  Selector/1 -> GLU Muscle/1(phiHip)
  HFL&HAM Muscles/3(TauHamKnee) -> Vector ConcatenateHip3/4, [RTauHamKnee], Vector ConcatenateKnee/1
  [RKneeStateOut] -> VAS Muscle/4(CLKneeState)
  [RphidphiKnee] -> Selector4/1
  [RphidphiKnee] -> Selector3/1
  [LonR] -> VAS Muscle/3(OLonCL)
  GLU Muscle/1(TauGlu) -> Vector ConcatenateHip/1, Vector ConcatenateHip3/1
  HFL&HAM Muscles/1(TauHFL) -> Vector ConcatenateHip/2, Vector ConcatenateHip3/2
  GAS Muscle/1(TauGasKnee) -> Vector ConcatenateKnee/3, Vector ConcatenateHip3/6
  [RphidphiAnkle] -> AnkleJoint right/1
  VAS Muscle/1(TauVas) -> Vector ConcatenateKnee/2, Vector ConcatenateHip3/5
  Selector6/1 -> GAS Muscle/2(phiAnkle)
  Selector3/1 -> VAS Muscle/1(phiKnee)
  SOL&TA Muscles/1(TauTA) -> Vector ConcatenateAnkle/2, Vector ConcatenateHip3/8
  Vector ConcatenateKnee/1 -> KneeJoint right/2
  Vector ConcatenateAnkle/1 -> Gain/1
  Selector7/1 -> SOL&TA Muscles/1(phiAnkle)
  SOL&TA Muscles/2(TauSOL) -> Vector ConcatenateHip3/9, Vector ConcatenateAnkle/3
  [LdxThighOut] -> VAS Muscle/2(OLdxThigh)
  Selector4/1 -> GAS Muscle/1(phiKnee)
  Selector1/1 -> HFL&HAM Muscles/1(phiHip)
  [RphidphiKnee] -> KneeJoint right/1
  Vector ConcatenateHip/1 -> HipJoint right/2
  GAS Muscle/2(TauGasAnkle) -> Vector ConcatenateAnkle/1, Vector ConcatenateHip3/7
  Gain/1 -> AnkleJoint right/2

== system nmm2DFullBody/Full Body Control (created using the nmc library)/Sensors1 ==
  Theta : Inport
  dTheta : Inport  Port=2
  LphidphiKnee : Inport  Port=3
  RphidphiKnee : Inport  Port=4
  LStance : Inport  Port=5
  RStance : Inport  Port=6
  Body Pitch loop delay : TransportDelay  DelayTime=ShortDelay
  Body Pitch loop delay. : TransportDelay  DelayTime=ShortDelay
  FootSensor : nmc/NMC Sensors/FootSensor
  KneeSensor : nmc/NMC Sensors/KneeSensor
  ThightSensor1 : nmc/NMC Sensors/ThightSensor
  ThightSensorSimulator : nmc/NMC Sensors/ThightSensorSimulator  Commented=on
  To Workspace : ToWorkspace  VariableName=L_GRF  SaveFormat=Timeseries  SampleTime=-1
  To Workspace1 : ToWorkspace  VariableName=R_GRF  SaveFormat=Timeseries  SampleTime=-1
  tag scope: LKneeStateOut=global, LdxThighOut=global, LonR=global, LstanceOut=global, RKneeStateOut=global, RdxThighOut=global, RonL=global, RstanceOut=global, ThetaDelayed=global, dThetaDelayed=global
  wires:
  Body Pitch loop delay/1 -> [dThetaDelayed]
  Body Pitch loop delay./1 -> [ThetaDelayed]
  dTheta/1 -> Body Pitch loop delay/1
  Theta/1 -> Body Pitch loop delay./1
  LStance/1 -> FootSensor/1
  RStance/1 -> FootSensor/2
  [RstanceOut] -> ThightSensorSimulator/2
  [LstanceOut] -> ThightSensorSimulator/1
  [leftGRF_vertical] -> To Workspace/1
  [rightGRF_vertical] -> To Workspace1/1
  ThightSensor1/2 -> [RdxThighOut]
  ThightSensor1/1 -> [LdxThighOut]
  FootSensor/4 -> [RonL]
  FootSensor/3 -> [LonR]
  FootSensor/2 -> [RstanceOut]
  FootSensor/1 -> [LstanceOut]
  KneeSensor/2 -> [RKneeStateOut]
  KneeSensor/1 -> [LKneeStateOut]
  RphidphiKnee/1 -> KneeSensor/2
  LphidphiKnee/1 -> KneeSensor/1
  [LdxThigh] -> ThightSensor1/1
  [RdxThigh] -> ThightSensor1/2

== system nmm2DFullBody/Full Body Control (created using the nmc library)/Subsystem ==
  Parameter variation : Subsystem

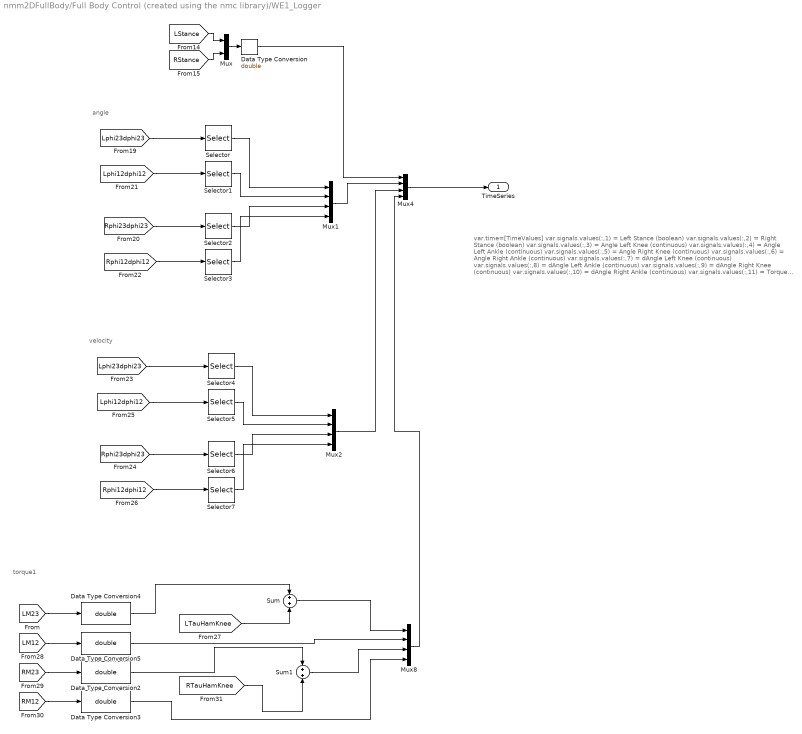
== system nmm2DFullBody/Full Body Control (created using the nmc library)/WE1_Logger ==
  note: torque1
  note: velocity
  note: angle
  note: var.time=[TimeValues]
      | var.signals.values(:,1) = Left Stance (boolean)
      | var.signals.values(:,2) = Right Stance (boolean)
      | var.signals.values(:,3) = Angle Left Knee (continuous)
      | var.signals.values(:,4) = Angle Left Ankle (continuous)
      | var.signals.values(:,5) = Angle Right Knee (continuous)
      | var.signals.values(:,6) = Angle Right Ankle (continuous)
      | var.signals.values(:,7) = dAngle Left Knee (continuous)
      | var.signals.values(:,8) = dAngle Left Ankle (continuous)
      | var.signals.values(:,9) = dAngle Right Knee (continuous)
      | var.signals.values(:,10) = dAngle Right Ankle (continuous)
      | var.signals.values(:,11) = Torque Left Knee (continuous)
      | var.signals.values(:,12) = Torque Left Ankle (continuous)
      | var.signals.values(:,13) = Torque Right Knee (continuous)
      | var.signals.values(:,14) = Torque Right Ankle (continuous)
      | var.signals.dimensions=[14]
  Data Type Conversion{,2..5} (5 alike) : DataTypeConversion  OutDataTypeStr=double
  Mux : Mux  Inputs=2
  Mux{1..2,4,8} (4 alike) : Mux
  Selector{,1..3} (4 alike) : Selector  InputPortWidth=2  IndexOptions=Index vector (dialog)  Indices=[1]  OutputSizes=1
  Selector{4..7} (4 alike) : Selector  InputPortWidth=2  IndexOptions=Index vector (dialog)  Indices=[2]  OutputSizes=1
  Sum : Sum
  Sum1 : Sum
  TimeSeries : Outport
  wires:
  [LM23] -> Data Type Conversion4/1
  [RM23] -> Data Type Conversion2/1
  [LM12] -> Data Type Conversion5/1
  Sum1/1 -> Mux8/3
  [RTauHamKnee] -> Sum1/2
  [Lphi23dphi23] -> Selector/1
  [Lphi12dphi12] -> Selector1/1
  [Rphi12dphi12] -> Selector3/1
  [Rphi23dphi23] -> Selector2/1
  [Lphi12dphi12] -> Selector5/1
  [Lphi23dphi23] -> Selector4/1
  [Rphi12dphi12] -> Selector7/1
  [Rphi23dphi23] -> Selector6/1
  Selector2/1 -> Mux1/3
  [LStance] -> Mux/1
  [RStance] -> Mux/2
  Selector/1 -> Mux1/1
  Selector1/1 -> Mux1/2
  Selector3/1 -> Mux1/4
  Selector4/1 -> Mux2/1
  Selector5/1 -> Mux2/2
  Selector6/1 -> Mux2/3
  Selector7/1 -> Mux2/4
  Mux/1 -> Data Type Conversion/1
  Mux1/1 -> Mux4/2
  Mux2/1 -> Mux4/3
  Mux8/1 -> Mux4/4
  Mux4/1 -> TimeSeries/1
  Data Type Conversion/1 -> Mux4/1
  [LTauHamKnee] -> Sum/2
  Data Type Conversion5/1 -> Mux8/2
  [RM12] -> Data Type Conversion3/1
  Data Type Conversion4/1 -> Sum/1
  Data Type Conversion3/1 -> Mux8/4
  Sum/1 -> Mux8/1
  Data Type Conversion2/1 -> Sum1/1

== system nmm2DFullBody/Noise Layer/Gaussian parameters ==
  mu : Inport
  sigma : Inport  Port=2
  tag scope: gaussianMean=global, gaussianStd=global
  wires:
  mu/1 -> [gaussianMean]
  sigma/1 -> [gaussianStd]

== system nmm2DFullBody/Noise Layer/Noise en right leg muscles ==
  gluteus : Inport
  hip flexor : Inport  Port=2
  hamstrings : Inport  Port=3
  vastus : Inport  Port=4
  gastrocnemius : Inport  Port=5
  soleus : Inport  Port=6
  tibialis : Inport  Port=7
  tag scope: RIGHT_GAS_STIM=global, RIGHT_GLU_STIM=global, RIGHT_HAM_STIM=global, RIGHT_HF_STIM=global, RIGHT_SOL_STIM=global, RIGHT_TA_STIM=global, RIGHT_VAS_STIM=global
  wires:
  gastrocnemius/1 -> [RIGHT_GAS_STIM]
  hamstrings/1 -> [RIGHT_HAM_STIM]
  hip flexor/1 -> [RIGHT_HF_STIM]
  soleus/1 -> [RIGHT_SOL_STIM]
  tibialis/1 -> [RIGHT_TA_STIM]
  gluteus/1 -> [RIGHT_GLU_STIM]
  vastus/1 -> [RIGHT_VAS_STIM]

== system nmm2DFullBody/Noise Layer/Noise on left leg group II afferent (muscle length) ==
  gluteus : Inport
  hip flexor : Inport  Port=2
  hamstrings : Inport  Port=3
  vastus : Inport  Port=4
  gastrocnemius : Inport  Port=5
  soleus : Inport  Port=6
  tibialis : Inport  Port=7
  tag scope: LEFT_GAS_LENGTH=global, LEFT_GLU_LENGTH=global, LEFT_HAM_LENGTH=global, LEFT_HF_LENGTH=global, LEFT_SOL_LENGTH=global, LEFT_TA_LENGTH=global, LEFT_VAS_LENGTH=global
  wires:
  gluteus/1 -> [LEFT_GLU_LENGTH]
  tibialis/1 -> [LEFT_TA_LENGTH]
  soleus/1 -> [LEFT_SOL_LENGTH]
  hamstrings/1 -> [LEFT_HAM_LENGTH]
  hip flexor/1 -> [LEFT_HF_LENGTH]
  gastrocnemius/1 -> [LEFT_GAS_LENGTH]
  vastus/1 -> [LEFT_VAS_LENGTH]

== system nmm2DFullBody/Noise Layer/Noise on left leg group II afferent (muscle length)1 ==
  note: nope
  note: nope
  gluteus : Inport
  hip flexor : Inport  Port=2
  hamstrings : Inport  Port=3
  vastus : Inport  Port=4
  gastrocnemius : Inport  Port=5
  soleus : Inport  Port=6
  tibialis : Inport  Port=7
  tag scope: LEFT_GAS_GOLGI=global, LEFT_GLU_GOLGI=global, LEFT_HAM_GOLGI=global, LEFT_HF_GOLGI=global, LEFT_SOL_GOLGI=global, LEFT_TA_GOLGI=global, LEFT_VAS_GOLGI=global
  wires:
  gluteus/1 -> [LEFT_GLU_GOLGI]
  tibialis/1 -> [LEFT_TA_GOLGI]
  soleus/1 -> [LEFT_SOL_GOLGI]
  hamstrings/1 -> [LEFT_HAM_GOLGI]
  hip flexor/1 -> [LEFT_HF_GOLGI]
  gastrocnemius/1 -> [LEFT_GAS_GOLGI]
  vastus/1 -> [LEFT_VAS_GOLGI]

== system nmm2DFullBody/Noise Layer/Noise on left leg group Ia afferent (muscle velocity) ==
  gluteus : Inport
  hip flexor : Inport  Port=2
  hamstrings : Inport  Port=3
  vastus : Inport  Port=4
  gastrocnemius : Inport  Port=5
  soleus : Inport  Port=6
  tibialis : Inport  Port=7
  tag scope: LEFT_GAS_VELOCITY=global, LEFT_GLU_VELOCITY=global, LEFT_HAM_VELOCITY=global, LEFT_HF_VELOCITY=global, LEFT_SOL_VELOCITY=global, LEFT_TA_VELOCITY=global, LEFT_VAS_VELOCITY=global
  wires:
  gluteus/1 -> [LEFT_GLU_VELOCITY]
  tibialis/1 -> [LEFT_TA_VELOCITY]
  soleus/1 -> [LEFT_SOL_VELOCITY]
  hamstrings/1 -> [LEFT_HAM_VELOCITY]
  hip flexor/1 -> [LEFT_HF_VELOCITY]
  gastrocnemius/1 -> [LEFT_GAS_VELOCITY]
  vastus/1 -> [LEFT_VAS_VELOCITY]

== system nmm2DFullBody/Noise Layer/Noise on left leg muscles ==
  gluteus : Inport
  hip flexor : Inport  Port=2
  hamstrings : Inport  Port=3
  vastus : Inport  Port=4
  gastrocnemius : Inport  Port=5
  soleus : Inport  Port=6
  tibialis : Inport  Port=7
  tag scope: LEFT_GAS_STIM=global, LEFT_GLU_STIM=global, LEFT_HAM_STIM=global, LEFT_HF_STIM=global, LEFT_SOL_STIM=global, LEFT_TA_STIM=global, LEFT_VAS_STIM=global
  wires:
  gluteus/1 -> [LEFT_GLU_STIM]
  tibialis/1 -> [LEFT_TA_STIM]
  soleus/1 -> [LEFT_SOL_STIM]
  hamstrings/1 -> [LEFT_HAM_STIM]
  hip flexor/1 -> [LEFT_HF_STIM]
  gastrocnemius/1 -> [LEFT_GAS_STIM]
  vastus/1 -> [LEFT_VAS_STIM]

== system nmm2DFullBody/Noise Layer/Noise on right leg group II afferent (muscle length) ==
  gluteus : Inport
  hip flexor : Inport  Port=2
  hamstrings : Inport  Port=3
  vastus : Inport  Port=4
  gastrocnemius : Inport  Port=5
  soleus : Inport  Port=6
  tibialis : Inport  Port=7
  tag scope: RIGHT_GAS_LENGTH=global, RIGHT_GLU_LENGTH=global, RIGHT_HAM_LENGTH=global, RIGHT_HF_LENGTH=global, RIGHT_SOL_LENGTH=global, RIGHT_TA_LENGTH=global, RIGHT_VAS_LENGTH=global
  wires:
  gastrocnemius/1 -> [RIGHT_GAS_LENGTH]
  hamstrings/1 -> [RIGHT_HAM_LENGTH]
  soleus/1 -> [RIGHT_SOL_LENGTH]
  tibialis/1 -> [RIGHT_TA_LENGTH]
  gluteus/1 -> [RIGHT_GLU_LENGTH]
  hip flexor/1 -> [RIGHT_HF_LENGTH]
  vastus/1 -> [RIGHT_VAS_LENGTH]

== system nmm2DFullBody/Noise Layer/Noise on right leg group II afferent (muscle length)1 ==
  gluteus : Inport
  hip flexor : Inport  Port=2
  hamstrings : Inport  Port=3
  vastus : Inport  Port=4
  gastrocnemius : Inport  Port=5
  soleus : Inport  Port=6
  tibialis : Inport  Port=7
  tag scope: RIGHT_GAS_GOLGI=global, RIGHT_GLU_GOLGI=global, RIGHT_HAM_GOLGI=global, RIGHT_HF_GOLGI=global, RIGHT_SOL_GOLGI=global, RIGHT_TA_GOLGI=global, RIGHT_VAS_GOLGI=global
  wires:
  gastrocnemius/1 -> [RIGHT_GAS_GOLGI]
  hamstrings/1 -> [RIGHT_HAM_GOLGI]
  soleus/1 -> [RIGHT_SOL_GOLGI]
  tibialis/1 -> [RIGHT_TA_GOLGI]
  gluteus/1 -> [RIGHT_GLU_GOLGI]
  hip flexor/1 -> [RIGHT_HF_GOLGI]
  vastus/1 -> [RIGHT_VAS_GOLGI]

== system nmm2DFullBody/Noise Layer/Noise on right leg group Ia afferent (muscle velocity) ==
  gluteus : Inport
  hip flexor : Inport  Port=2
  hamstrings : Inport  Port=3
  vastus : Inport  Port=4
  gastrocnemius : Inport  Port=5
  soleus : Inport  Port=6
  tibialis : Inport  Port=7
  tag scope: RIGHT_GAS_VELOCITY=global, RIGHT_GLU_VELOCITY=global, RIGHT_HAM_VELOCITY=global, RIGHT_HF_VELOCITY=global, RIGHT_SOL_VELOCITY=global, RIGHT_TA_VELOCITY=global, RIGHT_VAS_VELOCITY=global
  wires:
  gastrocnemius/1 -> [RIGHT_GAS_VELOCITY]
  hamstrings/1 -> [RIGHT_HAM_VELOCITY]
  hip flexor/1 -> [RIGHT_HF_VELOCITY]
  soleus/1 -> [RIGHT_SOL_VELOCITY]
  tibialis/1 -> [RIGHT_TA_VELOCITY]
  gluteus/1 -> [RIGHT_GLU_VELOCITY]
  vastus/1 -> [RIGHT_VAS_VELOCITY]

== system nmm2DFullBody/Noise Layer/gaussian noise source ==
  MATLAB Function : MATLAB Function  TreatAsAtomicUnit=on
  Selector : Selector  InputPortWidth=30  IndexOptions=Index vector (dialog)  Indices=1  OutputSizes=1
  Out1 : Outport
  wires:
  Selector/1 -> Out1/1
  [gaussianMean] -> MATLAB Function/1(mu)
  [gaussianStd] -> MATLAB Function/2(sigma)
  MATLAB Function/1(y) -> Selector/1

== system nmm2DFullBody/Noise Layer/gaussian noise source1 ==
  MATLAB Function : MATLAB Function  TreatAsAtomicUnit=on
  Selector : Selector  InputPortWidth=30  IndexOptions=Index vector (dialog)  Indices=1  OutputSizes=1
  Out1 : Outport
  wires:
  MATLAB Function/1(y) -> Selector/1
  [gaussianStd] -> MATLAB Function/2(sigma)
  [gaussianMean] -> MATLAB Function/1(mu)
  Selector/1 -> Out1/1

== system nmm2DFullBody/Body Mechanics Layer (from Geyer s 2010 model)/Left Ball Contact/Ground Friction Model ==
  note: Horizontal Ground Friction Model
  note: Vertical Ground Stiction Model
  dy [m] : Inport
  vy [m/s] : Inport  Port=2
  x [m] : Inport  Port=3
  vx [m/s] : Inport  Port=4
  Contact! : EnablePort  StatesWhenEnabling=reset
  Data Type Conversion : DataTypeConversion  OutDataTypeStr=double
  Friction Switch : Subsystem
  Gain3 : Gain  Gain=k_gy
  Gain4 : Gain  Gain=1/v_gy_max
  Logical Operator : Logic  Operator=NOT  AllPortsSameDT=off  OutDataTypeStr=boolean
  Mux1 : Mux  Inputs=2
  Sum1 : Sum
  X-Axis Kinetic Friction Model : Subsystem
  X-Axis Static Friction Model : Subsystem
  Y-Axis Ground Force : Fcn  Expr="- u(1)  *  (1-u(2)) * (u(2)<1)"
  Fy_Ground[N] : Outport  OutputWhenDisabled=reset  InitialOutput=0
      settings: AttributesFormatString=initial = '%<InitialOutput>'\nwhen disabled = '%<OutputWhenDisabled>'
  Fx_Friction [N] : Outport  Port=2  OutputWhenDisabled=reset  InitialOutput=0
      settings: AttributesFormatString=initial = '%<InitialOutput>'\nwhen\ndisabled\n'%<OutputWhenDisabled>'
  Stiction! : Outport  Port=3  OutputWhenDisabled=reset  InitialOutput=0
      settings: AttributesFormatString=initial = '%<InitialOutput>'\nwhen\ndisabled\n'%<OutputWhenDisabled>'
  wires:
  dy [m]/1 -> Gain3/1
  vy [m/s]/1 -> Gain4/1
  x [m]/1 -> X-Axis Static Friction Model/2(pos [m]), X-Axis Kinetic Friction Model/1(pos [m])
  vx [m/s]/1 -> X-Axis Static Friction Model/3(vel [m/s]), X-Axis Kinetic Friction Model/2(vel [m/s])
  X-Axis Kinetic Friction Model/1(posFP [m]) -> X-Axis Static Friction Model/4(posFP [m])
  X-Axis Kinetic Friction Model/3(F_Slide [N]) -> Sum1/2
  X-Axis Static Friction Model/1(F_Stick [N]) -> Sum1/1
  Sum1/1 -> Fx_Friction [N]/1
  Friction Switch/1(Stiction) -> X-Axis Static Friction Model/Enable, Logical Operator/1, Data Type Conversion/1
  X-Axis Static Friction Model/2(Sliding!) -> Friction Switch/1(Slide!)
  X-Axis Kinetic Friction Model/2(Stiction!) -> Friction Switch/2(Stick!)
  Logical Operator/1 -> X-Axis Kinetic Friction Model/Enable
  Data Type Conversion/1 -> Stiction!/1
  Mux1/1 -> Y-Axis Ground Force/1
  Gain3/1 -> Mux1/1
  Gain4/1 -> Mux1/2
  Y-Axis Ground Force/1 -> Fy_Ground[N]/1, X-Axis Static Friction Model/1(F_Normal [N]), X-Axis Kinetic Friction Model/3(F_Normal [N])
